simulink model "windEmulatorStep3"  (R2021a)
settings: Solver=ode4  StartTime=0.0  StopTime=inf  FixedStep=0.002  RelTol=1e-3
values from neighbouring files (symbols this model uses):
  ctrlModeSpeed = logical(false)    [initStep4.m]
  ctrlModeTorque = logical(true)    [initStep4.m]
  Dm_max = 40    [initStep4.m]
  EffMechMax = 0.93    [initStep4.m]
  EffMechMin = 0.79    [initStep4.m]
  FactorEff = psi2pa*cc2m3*(1/rev2rad)    (= 0.00109733470463)    [initStep4.m]
  genMaxTorque = 0.975*acs880RatedTorque    (= 78.48165)    [initStep4.m]
  Kdamping = -500    [OptimizationResultsLoad.m]
  Kpos = 0    [OptimizationResultsLoad.m]
  nPreDrop = 2900    [initStep4.m]
  nPreDropMin = 725    [initStep4.m]
  StatusWord = bitset(StatusWord,16)    [VFD_StatusWord.m]
  T = 4    [initStep4.m]
  wheelRadius = targetWaveBotVel/targetOmega    (= 0.00477464829276)    [initStep4.m]
undefined symbols (not defined in the file or in its folder): ACS880PILimLo, ACS880PILimUp, DiscIntNeverNeededParam, Gen_REF2_Max, Gen_SpeedScaling, minPressureRef, Motor_SpeedScaling, Motor_TorqueScaling, PressureControl, ratedTorque, rpm2rps, SpeedControl, speedScalingACS800, TorqueFieldbusScale, TorqueInputControl, TorqueRefMin
libraries: fl_lib x41, nesl_utility x24, slrealtimeethercatlib x21, sh_lib x16, cstblocks x4, simulink x3, pid_lib x3, sdl_lib x1, dspstat3 x1
(part 1 of 3)
settings Model: SimulationMode=external  Creator=SWEPT  LastModifiedBy=SWEPT
settings SolverCC: ConcurrentTasks=on  PositivePriorityOrder=on
settings OptimizationCC: BlockReduction=off  OptimizeBlockIOStorage=off
settings DebuggingCC: TasksWithSamePriorityMsg=none
settings HardwareCC: ProdBitPerLong=64  ProdLongLongMode=on  ProdHWDeviceType=Intel->x86-64 (Linux 64)
settings RTWCC: Description=Simulink Real-Time  SystemTargetFile=slrealtime.tlc  TemplateMakefile=slrealtime_default_tmf  RTWVerbose=off  Toolchain=Simulink Real-Time Toolchain  BuildConfiguration=Faster Runs  CodeExecutionProfiling=on  TargetLang=C++

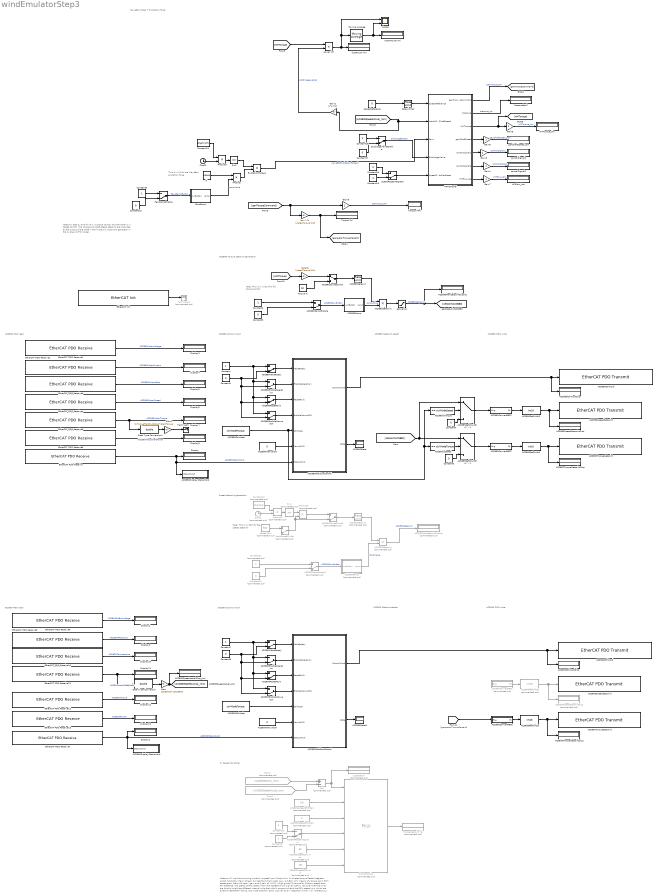
== system windEmulatorStep3 ==
  note: WaveBot Model + Excitation force
  note: PI Speed Controller
  note: Notes on PI:
      |
      | Input to summing junction is speed (rpm)
      | Output is in % of rated torque
      | Reset Integrator switch holds the I-Term at zero, but lets the P-Term pass.
      |
      | e.g., a P-Gain of 1 means 1% torque per 1 RPM speed error. Start with zero I gain and P gain of ~0.01, which gives 1% torque for 100rpm speed error.
      |
      | For reference, the speed control section from the ACS800 drive is given below. Not sure what the units are for this (might be different internal units than the % torque unit and the RPM speed unit, which are external (EtherCAT) facing. Also note that the I terms is given as an integration time in (s), whereas our integral term is a gain of the form Ki/s. The conversion should be: Ki = Kp/Ti. So to convert 2.5s with Kp = 10 gives Ki = 10/2.5 = 4.
      |
      | Jon undertook a re-tuning for the ACS880. This gave Kp = 5.84 and Ti = 0.33s. With this, Ki = 5.84/0.33 = 17.7.
      |
      | Start tuning Kp first, and then slowly bring Ki up to ~1-3 times Kp.
  note: Notes on Step 3:
      |
      | One drive is in torque control and the other is in speed control.
      |
      | The torque and shaft speed setpoint are produced as the output of the shaft in the hydraulic motor and generator in the hydraulic PTO model.
  note: ACS880 Torque setpoint generation
  note: ACS880 PDO write
  note: ASC880 Setpoint select
  note: Note: This is in units of % for torque control
  note: ACS880 Control Word
  note: ACS880 PDO read
  note: ACS800 PDO read
  note: ACS800 Control Word
  note: ASC800 Setpoint select
  note: ACS800 PDO write
  note: Speed setpoint generation
  note: Note: This is in RPM for the speed setpoint
  note: This is in (N) for the WaveBot excitation force
  ACS800ConvertREF1 : Subsystem  Commented=on  mask{EngineeringValue=Gen_SpeedScaling, FieldbusValue=20000}
      mask prompts: EngineeringValue "Engineering units nominal value:"; FieldbusValue "Fieldbus nominal value:"
  ACS800ConvertREF2 : Subsystem  mask{EngineeringValue=Gen_REF2_Max, FieldbusValue=10000}
      mask prompts: EngineeringValue "Engineering units nominal value:"; FieldbusValue "Fieldbus nominal value:"
  ACS800CtrlMode : Constant  Value=ctrlModeTorque  OutDataTypeStr=boolean
  ACS800CtrlWord : slrealtimeethercatlib/EtherCAT PDO Transmit  Priority=3  sig_name=Drive 2 (RECA-01 r2.07 and ACS800).RxPDO 1.ControlWord (Transparent)  sig_offset=384  sig_type=uint16  type_size=16  sig_dim=1  device_id=0  sample_time=0.002000
      settings: SourceProductBaseCode=XP
  ACS800CtrlWordDisp : Display
  ACS800DisplayStatusWord : Subsystem
  ACS800FieldbusControl : Subsystem
  ACS800ManualCW : Constant  Value=0  OutDataTypeStr=uint16
  ACS800Ramp : Stateflow chart  Commented=on  TreatAsAtomicUnit=on
  ACS800RampEnable : ManualSwitch  Commented=on  CurrentSetting=0
  ACS800RateLim : RateLimiter  Commented=on  RisingSlewLimit=10000  FallingSlewLimit=-10000  SampleTimeMode=inherited
  ACS800RawSetpointDisplay : Display  Commented=on
  ACS800Ref1Int16 : DataTypeConversion  Commented=on  OutDataTypeStr=int16
  ACS800Ref2Int16 : DataTypeConversion  OutDataTypeStr=int16
  ACS800ResetIntegrator : ManualSwitch  Commented=on  CurrentSetting=0
  ACS800Setpoint : Product  Commented=on
  ACS800SpeedCtrlIGain : Constant  Commented=on  Value=0
  ACS800SpeedCtrlLimLo : Constant  Commented=on  Value=-80
  ACS800SpeedCtrlLimUp : Constant  Commented=on  Value=80
  ACS800SpeedCtrlPGain : Constant  Commented=on  Value=0.6
  ACS800SpeedSetpoint : slrealtimeethercatlib/EtherCAT PDO Transmit  Priority=3  sig_name=Drive 2 (RECA-01 r2.07 and ACS800).RxPDO 1.REF1 (Speed)  sig_offset=400  sig_type=int16  type_size=16  sig_dim=1  device_id=0  sample_time=0.002000
      settings: SourceProductBaseCode=XP
  ACS800SpeedSetpointDisp : Display  Commented=on
  ACS800TorqueSetpoint : slrealtimeethercatlib/EtherCAT PDO Transmit  Priority=3  sig_name=Drive 2 (RECA-01 r2.07 and ACS800).RxPDO 1.REF2 (Torque)  sig_offset=416  sig_type=int16  type_size=16  sig_dim=1  device_id=0  sample_time=0.002000
      settings: SourceProductBaseCode=XP
  ACS800TorqueSetpointDisp : Display
  ACS880ConvertREF1 : Subsystem  mask{EngineeringValue=Motor_SpeedScaling, FieldbusValue=20000}
      mask prompts: EngineeringValue "Engineering units nominal value:"; FieldbusValue "Fieldbus nominal value:"
  ACS880ConvertREF2 : Subsystem  mask{EngineeringValue=Motor_TorqueScaling, FieldbusValue=10000}
      mask prompts: EngineeringValue "Engineering units nominal value:"; FieldbusValue "Fieldbus nominal value:"
  ACS880CtrlMode : Constant  Value=ctrlModeTorque  OutDataTypeStr=boolean
  ACS880CtrlWord : slrealtimeethercatlib/EtherCAT PDO Transmit  Priority=3  sig_name=Drive 1 (FECA-01 r1.31 and ACS880).RxPDO 1.ABB Drives Control Word  sig_offset=208  sig_type=uint16  type_size=16  sig_dim=1  device_id=0  sample_time=0.002000
      settings: SourceProductBaseCode=XP
  ACS880CtrlWordDisp : Display
  ACS880DisplayStatusWord : Subsystem
  ACS880FieldbusControl : Subsystem
  ACS880IsTorque : simulink/Logic and Bit Operations/Compare To Constant  relop===  const=ctrlModeSpeed  OutDataTypeStr=boolean
  ACS880ManualCW : Constant  Value=0  OutDataTypeStr=uint16
  ACS880Ramp : Stateflow chart  TreatAsAtomicUnit=on
  ACS880RampEnable : ManualSwitch  CurrentSetting=0
  ACS880RateLim : RateLimiter  RisingSlewLimit=10000  FallingSlewLimit=-10000  SampleTimeMode=inherited
  ACS880RawSetpointDisplay : Display
  ACS880Ref1Int16 : DataTypeConversion  OutDataTypeStr=int16
  ACS880Ref1Switch : Switch  Criteria=u2 > Threshold
  ACS880Ref2Int16 : DataTypeConversion  OutDataTypeStr=int16
  ACS880Ref2Switch : Switch  Criteria=u2 > Threshold
  ACS880Setpoint : Product
  ACS880SpeedActualDisp_rpm : Display
  ACS880SpeedSetpoint : slrealtimeethercatlib/EtherCAT PDO Transmit  Priority=3  sig_name=Drive 1 (FECA-01 r1.31 and ACS880).RxPDO 1.ABB Drives REF1  sig_offset=224  sig_type=int16  type_size=16  sig_dim=1  device_id=0  sample_time=0.002000
      settings: SourceProductBaseCode=XP
  ACS880SpeedSetpointDisp : Display
  ACS880TorqueSetpoint : slrealtimeethercatlib/EtherCAT PDO Transmit  Priority=3  sig_name=Drive 1 (FECA-01 r1.31 and ACS880).RxPDO 1.ABB Drives REF2  sig_offset=240  sig_type=int16  type_size=16  sig_dim=1  device_id=0  sample_time=0.002000
      settings: SourceProductBaseCode=XP
  ACS880TorqueSetpointDisp : Display
  ASC800EnableManualCW : ManualSwitch  CurrentSetting=0
  ASC800EnableOperation : ManualSwitch  CurrentSetting=0
  ASC800MakeReady : ManualSwitch  CurrentSetting=0
  ASC800ResetFault : ManualSwitch  CurrentSetting=0
  ASC800SourceSwitch : ManualSwitch  Commented=on  CurrentSetting=0
  ASC880EnableManualCW : ManualSwitch  CurrentSetting=0
  ASC880EnableOperation : ManualSwitch  CurrentSetting=0
  ASC880IsSpeed : simulink/Logic and Bit Operations/Compare To Constant  relop===  const=ctrlModeTorque  OutDataTypeStr=boolean
  ASC880MakeReady : ManualSwitch  CurrentSetting=0
  ASC880ResetFault : ManualSwitch  CurrentSetting=0
  ASC880SourceSwitch : ManualSwitch
  ASC880State : Display
  ASC880State1 : Display
  Add : Sum  Commented=on  Inputs=+-
  Clock1 : Clock  Commented=on
  Clock2 : Clock
  Constant{,2,5,7,16,19} (6 alike) : Constant
  Constant{1,3..4,6,8,15,17..18} (8 alike) : Constant  Value=0
  Constant10 : Constant  Commented=on  Value=0
  Constant11 : Constant  Commented=on
  Constant12 : Constant  Commented=on  Value=0
  Constant13 : Constant  Commented=on  Value=2*pi*0.2
  Constant14 : Constant  Value=2*pi*(1/T)
  Constant9 : Constant  Commented=on
  Data Type Conversion : DataTypeConversion  OutDataTypeStr=double
  Data Type Conversion1 : DataTypeConversion  OutDataTypeStr=double
  DischargeValveEnable : ManualSwitch  CurrentSetting=0
  Display{,1..13} (14 alike) : Display
  EtherCAT Init : slrealtimeethercatlib/EtherCAT Init  Priority=0  config_file=C:\Users\SWEPT\Desktop\Jorge\WIndTurbineEmulator\WindEmulatorFiles\ethercat\WindTurbineEmulator-03-24-2022.xml  device_id=0  pci_bus=0  pci_slot=0  pci_function=0  portnum=1  initstate=2  dctuning=0  enaDebug=0  enaDC=on  errLink=off  masterDbg=off  stateChgDbg=off  baseClock=off  masterCfg=off  logFile='c:\dbglog.txt'  sample_time=0.002000  DCMode=0
      settings: SourceProductBaseCode=XP
  EtherCAT PDO Receive : slrealtimeethercatlib/EtherCAT PDO Receive  Priority=2  sig_name=Drive 1 (FECA-01 r1.31 and ACS880).TxPDO 1.ABB Drives Status Word  sig_offset=208  sig_type=uint16  type_size=16  sig_dim=1  device_id=0  sample_time=0.002000
      settings: SourceProductBaseCode=XP
  EtherCAT PDO Receive1 : slrealtimeethercatlib/EtherCAT PDO Receive  Priority=2  sig_name=Drive 1 (FECA-01 r1.31 and ACS880).TxPDO 6.Calculated motor voltage  sig_offset=304  sig_type=int16  type_size=16  sig_dim=1  device_id=0  sample_time=0.002000
      settings: SourceProductBaseCode=XP
  EtherCAT PDO Receive10 : slrealtimeethercatlib/EtherCAT PDO Receive  Priority=2  sig_name=Drive 2 (RECA-01 r2.07 and ACS800).TxPDO 1.Converter Temperature  sig_offset=496  sig_type=int16  type_size=16  sig_dim=1  device_id=0  sample_time=0.002000
      settings: SourceProductBaseCode=XP
  EtherCAT PDO Receive11 : slrealtimeethercatlib/EtherCAT PDO Receive  Priority=2  sig_name=Drive 2 (RECA-01 r2.07 and ACS800).TxPDO 1.Actual Feedback (Transparent)  sig_offset=400  sig_type=int16  type_size=16  sig_dim=1  device_id=0  sample_time=0.002000
      settings: SourceProductBaseCode=XP
  EtherCAT PDO Receive12 : slrealtimeethercatlib/EtherCAT PDO Receive  Priority=2  sig_name=Drive 2 (RECA-01 r2.07 and ACS800).TxPDO 1.Torque  sig_offset=432  sig_type=int16  type_size=16  sig_dim=1  device_id=0  sample_time=0.002000
      settings: SourceProductBaseCode=XP
  EtherCAT PDO Receive13 : slrealtimeethercatlib/EtherCAT PDO Receive  Priority=2  sig_name=Drive 2 (RECA-01 r2.07 and ACS800).TxPDO 1.Power  sig_offset=448  sig_type=int16  type_size=16  sig_dim=1  device_id=0  sample_time=0.002000
      settings: SourceProductBaseCode=XP
  EtherCAT PDO Receive2 : slrealtimeethercatlib/EtherCAT PDO Receive  Priority=2  sig_name=Drive 1 (FECA-01 r1.31 and ACS880).TxPDO 6.Measured motor current  sig_offset=288  sig_type=int16  type_size=16  sig_dim=1  device_id=0  sample_time=0.002000
      settings: SourceProductBaseCode=XP
  EtherCAT PDO Receive3 : slrealtimeethercatlib/EtherCAT PDO Receive  Priority=2  sig_name=Drive 1 (FECA-01 r1.31 and ACS880).TxPDO 6.Estimated output frequency  sig_offset=272  sig_type=int16  type_size=16  sig_dim=1  device_id=0  sample_time=0.002000
      settings: SourceProductBaseCode=XP
  EtherCAT PDO Receive4 : slrealtimeethercatlib/EtherCAT PDO Receive  Priority=2  sig_name=Drive 1 (FECA-01 r1.31 and ACS880).TxPDO 6.Motor speed used  sig_offset=256  sig_type=int16  type_size=16  sig_dim=1  device_id=0  sample_time=0.002000
      settings: SourceProductBaseCode=XP
  EtherCAT PDO Receive5 : slrealtimeethercatlib/EtherCAT PDO Receive  Priority=2  sig_name=Drive 1 (FECA-01 r1.31 and ACS880).TxPDO 6.Motor torque  sig_offset=320  sig_type=int16  type_size=16  sig_dim=1  device_id=0  sample_time=0.002000
      settings: SourceProductBaseCode=XP
  EtherCAT PDO Receive6 : slrealtimeethercatlib/EtherCAT PDO Receive  Priority=2  sig_name=Drive 1 (FECA-01 r1.31 and ACS880).TxPDO 6.Estimated motor shaft power  sig_offset=336  sig_type=int16  type_size=16  sig_dim=1  device_id=0  sample_time=0.002000
      settings: SourceProductBaseCode=XP
  EtherCAT PDO Receive7 : slrealtimeethercatlib/EtherCAT PDO Receive  Priority=2  sig_name=Drive 2 (RECA-01 r2.07 and ACS800).TxPDO 1.Main StatusWord (Transparent)  sig_offset=384  sig_type=uint16  type_size=16  sig_dim=1  device_id=0  sample_time=0.002000
      settings: SourceProductBaseCode=XP
  EtherCAT PDO Receive8 : slrealtimeethercatlib/EtherCAT PDO Receive  Priority=2  sig_name=Drive 2 (RECA-01 r2.07 and ACS800).TxPDO 1.DC Bus Voltage  sig_offset=480  sig_type=int16  type_size=16  sig_dim=1  device_id=0  sample_time=0.002000
      settings: SourceProductBaseCode=XP
  EtherCAT PDO Receive9 : slrealtimeethercatlib/EtherCAT PDO Receive  Priority=2  sig_name=Drive 2 (RECA-01 r2.07 and ACS800).TxPDO 1.Frequency  sig_offset=464  sig_type=int16  type_size=16  sig_dim=1  device_id=0  sample_time=0.002000
      settings: SourceProductBaseCode=XP
  ExcitationForce_N : Product
  FexcRamp : Stateflow chart  TreatAsAtomicUnit=on
  FexcRampEnable : ManualSwitch  CurrentSetting=0
  From1 : From  Commented=on  GotoTag=ACS800SpeedActual_rpm
  From2 : From  Commented=on  GotoTag=speedSetpoint_rpm
  Gain : Gain  Gain=speedScalingACS800
  Gain1 : Gain  Gain=(1/TorqueFieldbusScale)*ratedTorque
  Gain2 : Gain  Gain=(2*pi)/60
  Gain{3..8} (6 alike) : Gain
  HMFlow_lpm : Display
  HMTorque_Nm : Display
  HPTOModel : Subsystem
  Moving Average : dspstat3/Moving Average  Method=Sliding window  ForgettingFactorPort=off  SpecifyWindowLength=on  WindowLength=20*500  ForgettingFactor=0.9  SimulateUsing=Code generation
  N : Constant  Value=15000
  "Nm -> %" : Gain  Gain=1/ratedTorque*100
  Nmto% : Gain  Gain=1/ratedTorque*100
  PID Controller : pid_lib/PID Controller  Commented=on  Controller=PI  Form=Parallel  TimeDomain=Discrete-time  UseExternalTs=off  SampleTime=-1  IntegratorMethod=Forward Euler  FilterMethod=Forward Euler  ControllerParametersSource=external  P=1  I=1  D=0  UseFilter=on  N=100  TunerSelectOption=Transfer Function Based (PID Tuner App)  InitialConditionSource=internal  InitialConditionForIntegrator=0  InitialConditionForFilter=0  DifferentiatorICPrevScaledInput=0  ExternalReset=level  TrackingMode=off  Kt=1  LimitOutput=on  SatLimitsSource=external  UpperSaturationLimit=inf  LowerSaturationLimit=-inf  LinearizeAsGain=on  AntiWindupMode=clamping  Kb=1  POutMin=[]  POutMax=[]  IOutMin=[]  IOutMax=[]  DOutMin=[]  DOutMax=[]  NOutMin=[]  NOutMax=[]  SumOutMin=[]  SumOutMax=[]  SaturationOutMin=[]  SaturationOutMax=[]  PParamMin=[]  PParamMax=[]  IParamMin=[]  IParamMax=[]  DParamMin=[]  DParamMax=[]  NParamMin=[]  NParamMax=[]  KbParamMin=[]  KbParamMax=[]  KtParamMin=[]  KtParamMax=[]  KbOutMin=[]  KbOutMax=[]  KtOutMin=[]  KtOutMax=[]  IntegratorOutMin=[]  IntegratorOutMax=[]  FilterOutMin=[]  FilterOutMax=[]  SumI1OutMin=[]  SumI1OutMax=[]  SumI2OutMin=[]  SumI2OutMax=[]  SumI3OutMin=[]  SumI3OutMax=[]  SumI4OutMin=[]  SumI4OutMax=[]  SumDOutMin=[]  SumDOutMax=[]  DifferentiatorOutMin=[]  DifferentiatorOutMax=[]  FilterDiffOutCoefMin=[]  FilterDiffOutCoefMax=[]  ReciprocalOutMin=[]  ReciprocalOutMax=[]  SumDenOutMin=[]  SumDenOutMax=[]  SumNumOutMin=[]  SumNumOutMax=[]  DivideOutMin=[]  DivideOutMax=[]  UdiffTsProdOutMin=[]  UdiffTsProdOutMax=[]  NTsProdOutMin=[]  NTsProdOutMax=[]  UintegralTsProdOutMin=[]  UintegralTsProdOutMax=[]  UngainTsProdOutMin=[]  UngainTsProdOutMax=[]  IntegratorContinuousStateAttributes=''  IntegratorStateMustResolveToSignalObject=off  IntegratorRTWStateStorageClass=Auto  FilterContinuousStateAttributes=''  FilterStateMustResolveToSignalObject=off  FilterRTWStateStorageClass=Auto  ParallelPVariant=ExternalParameters  IdealPVariant=Disabled  IVariant=ExternalParameters  DVariant=Disabled  IntegratorVariant=Discrete  SatVariant=External  AWVariant=DiscClampingParallel  PCopyVariant=Disabled  TRVariant=Disabled  FdbkBlocksVariant=Forward  IdealPFdbkVariant=Disabled  SatFdbkVariant=Disabled  DerivativeFilterVariant=Disabled  NVariant=Disabled  NCopyVariant=Disabled_SignalSpec  FilterICVariant=Disabled  IntegratorICVariant=InternalICs  ExternalResetVariant=ExternalReset  TRSumVariant=Passthrough  SumFdbkVariant=Disabled  SumVariant=Sum_PI  TsampFilterVariant=InternalTs  TsampNgainVariant=Passthrough  TsampIntegralVariant=Passthrough  ExternalSaturationOutDataTypeStr=Inherit: Same as second input
  Pressure[psi] : Display
  Product : Product
  Product2 : Product  Commented=on
  Product3 : Product  Commented=on
  Product4 : Product
  Rate Limiter : RateLimiter  RisingSlewLimit=50  FallingSlewLimit=-50  SampleTimeMode=inherited
  Saturation : Saturate  UpperLimit=ACS880PILimUp  LowerLimit=ACS880PILimLo
  Scope : Scope  NumInputPorts=2
  Sin1 : Trigonometry  Commented=on
  Sin2 : Trigonometry
  Speed RPM : Constant  Commented=on  Value=500
  SpeedError : Display  Commented=on
  SpeedReference : Constant  Value=0
  SpeedResetIntegrator : ManualSwitch  CurrentSetting=0
  Terminator : Terminator
  Terminator1 : Terminator  Commented=on
  Torque % : Constant  Value=10
  Torque (%) : Display
  Torque (Nm) : Display
  TorqueSetpoint (%) : Display  Commented=on
  controlSignal1 : Display
  controlSignal2 : Display
  dispPower (W) : Display
  genShaftSpeed_rpm : Display
  meanPower (W) : Display
  power (W) : Product
  shaftSpeedSwitch : ManualSwitch  Commented=on  CurrentSetting=0
  wires:
  EtherCAT Init/1 -> Terminator1/1
  ASC880EnableOperation/1 -> ACS880FieldbusControl/2(EnableOperation)
  ACS880ManualCW/1 -> ACS880FieldbusControl/6(ManualCW)
  ASC880ResetFault/1 -> ACS880FieldbusControl/3(ResetFault)
  ASC880MakeReady/1 -> ACS880FieldbusControl/1(MakeReady)
  ASC880EnableManualCW/1 -> ACS880FieldbusControl/4(EnableManualCW)
  Constant1/1 -> ASC880EnableManualCW/2, ASC880ResetFault/2, ASC880EnableOperation/2, ASC880MakeReady/2
  Constant/1 -> ASC880EnableManualCW/1, ASC880ResetFault/1, ASC880EnableOperation/1, ASC880MakeReady/1
  ACS880FieldbusControl/2(state) -> ASC880State/1
  EtherCAT PDO Receive1/1 -> Display3/1  "ACS880MotorVoltage"
  EtherCAT PDO Receive2/1 -> Display4/1  "ACS880MotorCurrent"
  EtherCAT PDO Receive3/1 -> Display5/1  "ACS880OutputFreq"
  EtherCAT PDO Receive4/1 -> Display6/1  "ACS880MotorSpeed"
  EtherCAT PDO Receive5/1 -> Display7/1, Data Type Conversion1/1  "ACS880MotorTorque"
  EtherCAT PDO Receive6/1 -> Display8/1  "ACS880MotorShaftPower"
  ACS880RampEnable/1 -> ACS880Ramp/1(runButton)  "ACS880RunButton"
  Constant3/1 -> ACS880RampEnable/2
  Constant2/1 -> ACS880RampEnable/1
  ACS880Ramp/1(ramp) -> ACS880Setpoint/2  "rampValue"
  ACS880Setpoint/1 -> Saturation/1
  ACS880RateLim/1 -> ACS880Setpoint/1
  ACS880ConvertREF1/1(Fb) -> ACS880Ref1Int16/1
  ACS880Ref1Int16/1 -> ACS880SpeedSetpointDisp/1, ACS880SpeedSetpoint/1
  ACS880Ref2Int16/1 -> ACS880TorqueSetpoint/1, ACS880TorqueSetpointDisp/1
  ACS880ConvertREF2/1(Fb) -> ACS880Ref2Int16/1
  ACS880CtrlMode/1 -> ACS880FieldbusControl/5(CtrlMode), ACS880IsTorque/1, ASC880IsSpeed/1
  EtherCAT PDO Receive/1 -> ACS880DisplayStatusWord/1(StatusWord), ACS880FieldbusControl/7(StatusWord), Display/1  "ACS880StatusWord"
  ACS880IsTorque/1 -> ACS880Ref1Switch/2
  [setpointACS880] -> ACS880Ref1Switch/1, ACS880Ref2Switch/1
  Constant4/1 -> ACS880Ref1Switch/3
  ASC880IsSpeed/1 -> ACS880Ref2Switch/2
  Constant6/1 -> ACS880Ref2Switch/3
  ACS880FieldbusControl/1(ControlWord) -> ACS880CtrlWordDisp/1, ACS880CtrlWord/1
  ACS880Ref1Switch/1 -> ACS880ConvertREF1/1(Eng)
  ACS880Ref2Switch/1 -> ACS880ConvertREF2/1(Eng)
  Torque %/1 -> ASC880SourceSwitch/2
  ASC880SourceSwitch/1 -> ACS880RateLim/1
  EtherCAT PDO Receive13/1 -> Display13/1  "ACS800Power"
  EtherCAT PDO Receive11/1 -> Data Type Conversion/1, Display11/1  "ACS800ActualFeedback"
  EtherCAT PDO Receive9/1 -> Display9/1  "ACS800Frequency"
  EtherCAT PDO Receive12/1 -> Display12/1  "ACS800Torque"
  EtherCAT PDO Receive10/1 -> Display10/1  "ACS800Temperature"
  EtherCAT PDO Receive8/1 -> Display2/1  "ACS800DcBusVoltage"
  ASC800EnableOperation/1 -> ACS800FieldbusControl/2(EnableOperation)
  ASC800ResetFault/1 -> ACS800FieldbusControl/3(ResetFault)
  ACS800ManualCW/1 -> ACS800FieldbusControl/6(ManualCW)
  EtherCAT PDO Receive7/1 -> ACS800DisplayStatusWord/1(StatusWord), ACS800FieldbusControl/7(StatusWord), Display1/1  "ACS800StatusWord"
  Constant7/1 -> ASC800EnableManualCW/1, ASC800ResetFault/1, ASC800EnableOperation/1, ASC800MakeReady/1
  ACS800FieldbusControl/2(state) -> ASC880State1/1
  Constant8/1 -> ASC800EnableManualCW/2, ASC800ResetFault/2, ASC800EnableOperation/2, ASC800MakeReady/2
  ASC800MakeReady/1 -> ACS800FieldbusControl/1(MakeReady)
  ASC800EnableManualCW/1 -> ACS800FieldbusControl/4(EnableManualCW)
  ACS800CtrlMode/1 -> ACS800FieldbusControl/5(CtrlMode)
  ACS800ConvertREF2/1(Fb) -> ACS800Ref2Int16/1
  ACS800Ref2Int16/1 -> ACS800TorqueSetpointDisp/1, ACS800TorqueSetpoint/1
  ACS800Ref1Int16/1 -> ACS800SpeedSetpoint/1, ACS800SpeedSetpointDisp/1
  ACS800ConvertREF1/1(Fb) -> ACS800Ref1Int16/1
  ACS800FieldbusControl/1(ControlWord) -> ACS800CtrlWordDisp/1, ACS800CtrlWord/1
  PID Controller/1 -> TorqueSetpoint (%)/1
  ASC800SourceSwitch/1 -> ACS800RateLim/1
  Product3/1 -> ASC800SourceSwitch/1
  Sin1/1 -> Product3/1
  ACS800RateLim/1 -> ACS800Setpoint/1
  ACS800Setpoint/1 -> ACS800RawSetpointDisplay/1  "ACS800Setpoint"
  Constant13/1 -> Product2/1
  Product2/1 -> Sin1/1
  Clock1/1 -> Product2/2
  ACS800Ramp/1(ramp) -> ACS800Setpoint/2  "rampValue"
  Constant11/1 -> ACS800RampEnable/1
  Constant12/1 -> ACS800RampEnable/2
  ACS800RampEnable/1 -> ACS800Ramp/1(runButton)  "ACS800RunButton"
  Gain/1 -> ACS880SpeedActualDisp_rpm/1, [ACS800SpeedActual_rpm]
  From2/1 -> Add/1
  From1/1 -> Add/2
  Add/1 -> SpeedError/1, PID Controller/1
  ACS800SpeedCtrlPGain/1 -> PID Controller/2
  ACS800SpeedCtrlIGain/1 -> PID Controller/3
  ACS800ResetIntegrator/1 -> PID Controller/4
  Constant9/1 -> ACS800ResetIntegrator/2
  Constant10/1 -> ACS800ResetIntegrator/1
  Data Type Conversion/1 -> Gain/1
  ACS800SpeedCtrlLimUp/1 -> PID Controller/5
  ACS800SpeedCtrlLimLo/1 -> PID Controller/6
  Product4/1 -> Sin2/1
  Clock2/1 -> Product4/2
  Constant14/1 -> Product4/1
  ExcitationForce_N/1 -> HPTOModel/3(Fexc)  "waveBotExcitationForce_N"
  [genTorqueCommand] -> Gain5/1, "Nm -> %"/1
  Sin2/1 -> ExcitationForce_N/1
  power (W)/1 -> Scope/1, Moving Average/1, dispPower (W)/1
  [ACS800SpeedActual_rpm] -> Gain2/1, HPTOModel/2(ActualGenShaftSpeed)
  Moving Average/1 -> Scope/2, meanPower (W)/1
  Saturation/1 -> [setpointACS880], ACS880RawSetpointDisplay/1  "ACS880Setpoint"
  Data Type Conversion1/1 -> Gain1/1
  HPTOModel/1(genTorqueCommand) -> [genTorqueCommand]  "genTorque_Nm"
  Constant5/1 -> FexcRampEnable/1
  Constant15/1 -> FexcRampEnable/2
  FexcRampEnable/1 -> FexcRamp/1(runButton)  "FexcRampButton"
  FexcRamp/1(ramp) -> Product/2  "rampValue"
  N/1 -> Product/1
  Product/1 -> ExcitationForce_N/2
  Speed RPM/1 -> shaftSpeedSwitch/1
  shaftSpeedSwitch/1 -> ASC800SourceSwitch/2, Product3/2
  HPTOModel/2(Pressure) -> Pressure[psi]/1  "pressure_psi"
  DischargeValveEnable/1 -> HPTOModel/4(DischargeValve)  "DischargeButton"
  Constant16/1 -> DischargeValveEnable/1
  Constant17/1 -> DischargeValveEnable/2
  Constant19/1 -> SpeedResetIntegrator/2
  Constant18/1 -> SpeedResetIntegrator/1
  SpeedResetIntegrator/1 -> HPTOModel/5(SpeedControllerReset)
  [generatorTorquePercent] -> ACS800ConvertREF2/1(Eng)
  "Nm -> %"/1 -> [generatorTorquePercent], Torque (%)/1
  SpeedReference/1 -> Rate Limiter/1
  HPTOModel/3(HMTorque) -> Gain6/1, [HMTorque]
  HPTOModel/4(genShaftSpeed) -> Gain8/1
  [HMTorque] -> Nmto%/1
  Nmto%/1 -> ASC880SourceSwitch/1
  Gain2/1 -> power (W)/2  "ptoOmega_radps"
  Gain1/1 -> Terminator/1
  HPTOModel/5(controlSignal1) -> Gain3/1
  HPTOModel/6(controlSignal2) -> Gain4/1
  HPTOModel/7(HMFlow_lps) -> Gain7/1
  Rate Limiter/1 -> HPTOModel/1(SpeedReference)
  Gain3/1 -> controlSignal1/1  "controlSignal1"
  Gain4/1 -> controlSignal2/1  "controlSignal2"
  Gain5/1 -> Torque (Nm)/1  "ptoTorque_Nm"
  Gain6/1 -> HMTorque_Nm/1  "HMTorque_Nm"
  [HMTorque] -> power (W)/1
  Gain7/1 -> HMFlow_lpm/1  "HMFlow_lpm"
  Gain8/1 -> genShaftSpeed_rpm/1  "genShaftSpeed_rpm"

== system windEmulatorStep3/ACS800ConvertREF1 ==
  Eng : Inport
  Constant EngineeringValue : Constant  Value=EngineeringValue
  Constant FieldbusValue : Constant  Value=FieldbusValue
  Product : Product  Inputs=**/
  Fb : Outport
  wires:
  Constant EngineeringValue/1 -> Product/3
  Constant FieldbusValue/1 -> Product/2
  Eng/1 -> Product/1
  Product/1 -> Fb/1

== system windEmulatorStep3/ACS800ConvertREF2 ==
  Eng : Inport
  Constant EngineeringValue : Constant  Value=EngineeringValue
  Constant FieldbusValue : Constant  Value=FieldbusValue
  Product : Product  Inputs=**/
  Fb : Outport
  wires:
  Constant EngineeringValue/1 -> Product/3
  Constant FieldbusValue/1 -> Product/2
  Eng/1 -> Product/1
  Product/1 -> Fb/1

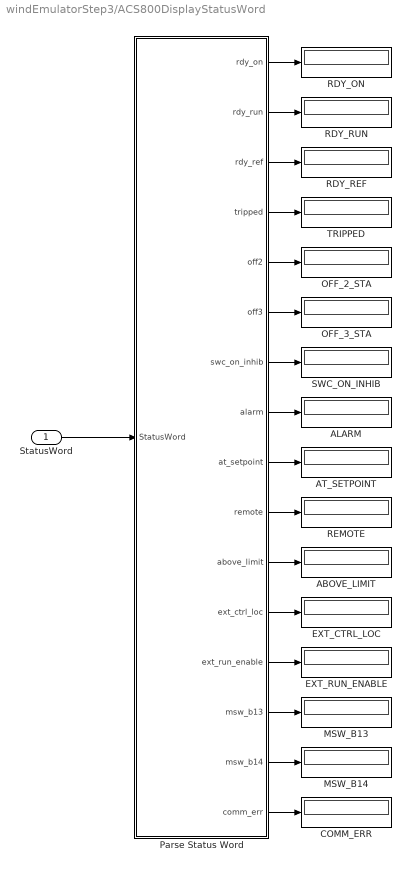
== system windEmulatorStep3/ACS800DisplayStatusWord ==
  StatusWord : Inport
  ABOVE_LIMIT : Display
  ALARM : Display
  AT_SETPOINT : Display
  COMM_ERR : Display
  EXT_CTRL_LOC : Display
  EXT_RUN_ENABLE : Display
  MSW_B13 : Display
  MSW_B14 : Display
  OFF_2_STA : Display
  OFF_3_STA : Display
  Parse Status Word : MATLAB Function  TreatAsAtomicUnit=on
  RDY_ON : Display
  RDY_REF : Display
  RDY_RUN : Display
  REMOTE : Display
  SWC_ON_INHIB : Display
  TRIPPED : Display
  wires:
  Parse Status Word/11(above_limit) -> ABOVE_LIMIT/1
  Parse Status Word/3(rdy_ref) -> RDY_REF/1
  Parse Status Word/16(comm_err) -> COMM_ERR/1
  Parse Status Word/15(msw_b14) -> MSW_B14/1
  Parse Status Word/14(msw_b13) -> MSW_B13/1
  Parse Status Word/8(alarm) -> ALARM/1
  Parse Status Word/2(rdy_run) -> RDY_RUN/1
  Parse Status Word/5(off2) -> OFF_2_STA/1
  Parse Status Word/12(ext_ctrl_loc) -> EXT_CTRL_LOC/1
  Parse Status Word/4(tripped) -> TRIPPED/1
  Parse Status Word/6(off3) -> OFF_3_STA/1
  Parse Status Word/1(rdy_on) -> RDY_ON/1
  Parse Status Word/9(at_setpoint) -> AT_SETPOINT/1
  Parse Status Word/7(swc_on_inhib) -> SWC_ON_INHIB/1
  Parse Status Word/13(ext_run_enable) -> EXT_RUN_ENABLE/1
  Parse Status Word/10(remote) -> REMOTE/1
  StatusWord/1 -> Parse Status Word/1(StatusWord)

== system windEmulatorStep3/ACS800FieldbusControl ==
  MakeReady : Inport
  EnableOperation : Inport  Port=2
  ResetFault : Inport  Port=3
  EnableManualCW : Inport  Port=4
  CtrlMode : Inport  Port=5
  ManualCW : Inport  Port=6  OutDataTypeStr=uint16
  StatusWord : Inport  Port=7
  ABB Fieldbus Control : Stateflow chart  TreatAsAtomicUnit=on
  Switch1 : Switch  Criteria=u2 ~= 0
  ControlWord : Outport
  state : Outport  Port=2
  wires:
  EnableOperation/1 -> ABB Fieldbus Control/1(EnableOperation)
  ManualCW/1 -> Switch1/1
  MakeReady/1 -> ABB Fieldbus Control/2(MakeReady)
  ABB Fieldbus Control/1(ControlWord) -> Switch1/3
  ResetFault/1 -> ABB Fieldbus Control/3(ResetFault)
  Switch1/1 -> ControlWord/1
  EnableManualCW/1 -> Switch1/2
  StatusWord/1 -> ABB Fieldbus Control/4(StatusWord)
  ABB Fieldbus Control/2(state) -> state/1
  CtrlMode/1 -> ABB Fieldbus Control/5(cwEXT_CTRL_LOC)

== system windEmulatorStep3/ACS880ConvertREF1 ==
  Eng : Inport
  Constant EngineeringValue : Constant  Value=EngineeringValue
  Constant FieldbusValue : Constant  Value=FieldbusValue
  Product : Product  Inputs=**/
  Fb : Outport
  wires:
  Product/1 -> Fb/1
  Eng/1 -> Product/1
  Constant FieldbusValue/1 -> Product/2
  Constant EngineeringValue/1 -> Product/3

== system windEmulatorStep3/ACS880ConvertREF2 ==
  Eng : Inport
  Constant EngineeringValue : Constant  Value=EngineeringValue
  Constant FieldbusValue : Constant  Value=FieldbusValue
  Product : Product  Inputs=**/
  Fb : Outport
  wires:
  Product/1 -> Fb/1
  Eng/1 -> Product/1
  Constant FieldbusValue/1 -> Product/2
  Constant EngineeringValue/1 -> Product/3

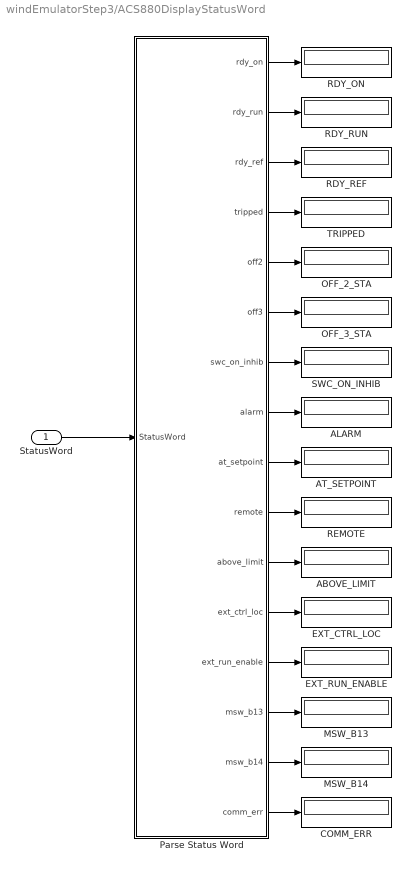
== system windEmulatorStep3/ACS880DisplayStatusWord ==
  StatusWord : Inport
  ABOVE_LIMIT : Display
  ALARM : Display
  AT_SETPOINT : Display
  COMM_ERR : Display
  EXT_CTRL_LOC : Display
  EXT_RUN_ENABLE : Display
  MSW_B13 : Display
  MSW_B14 : Display
  OFF_2_STA : Display
  OFF_3_STA : Display
  Parse Status Word : MATLAB Function  TreatAsAtomicUnit=on
  RDY_ON : Display
  RDY_REF : Display
  RDY_RUN : Display
  REMOTE : Display
  SWC_ON_INHIB : Display
  TRIPPED : Display
  wires:
  Parse Status Word/11(above_limit) -> ABOVE_LIMIT/1
  Parse Status Word/3(rdy_ref) -> RDY_REF/1
  Parse Status Word/16(comm_err) -> COMM_ERR/1
  Parse Status Word/15(msw_b14) -> MSW_B14/1
  Parse Status Word/14(msw_b13) -> MSW_B13/1
  Parse Status Word/8(alarm) -> ALARM/1
  Parse Status Word/2(rdy_run) -> RDY_RUN/1
  Parse Status Word/5(off2) -> OFF_2_STA/1
  Parse Status Word/12(ext_ctrl_loc) -> EXT_CTRL_LOC/1
  Parse Status Word/4(tripped) -> TRIPPED/1
  Parse Status Word/6(off3) -> OFF_3_STA/1
  Parse Status Word/1(rdy_on) -> RDY_ON/1
  Parse Status Word/9(at_setpoint) -> AT_SETPOINT/1
  Parse Status Word/7(swc_on_inhib) -> SWC_ON_INHIB/1
  Parse Status Word/13(ext_run_enable) -> EXT_RUN_ENABLE/1
  Parse Status Word/10(remote) -> REMOTE/1
  StatusWord/1 -> Parse Status Word/1(StatusWord)

== system windEmulatorStep3/ACS880FieldbusControl ==
  MakeReady : Inport
  EnableOperation : Inport  Port=2
  ResetFault : Inport  Port=3
  EnableManualCW : Inport  Port=4
  CtrlMode : Inport  Port=5
  ManualCW : Inport  Port=6  OutDataTypeStr=uint16
  StatusWord : Inport  Port=7
  ABB Fieldbus Control : Stateflow chart  TreatAsAtomicUnit=on
  Switch1 : Switch  Criteria=u2 ~= 0
  ControlWord : Outport
  state : Outport  Port=2
  wires:
  EnableOperation/1 -> ABB Fieldbus Control/1(EnableOperation)
  ManualCW/1 -> Switch1/1
  MakeReady/1 -> ABB Fieldbus Control/2(MakeReady)
  ABB Fieldbus Control/1(ControlWord) -> Switch1/3
  ResetFault/1 -> ABB Fieldbus Control/3(ResetFault)
  Switch1/1 -> ControlWord/1
  EnableManualCW/1 -> Switch1/2
  StatusWord/1 -> ABB Fieldbus Control/4(StatusWord)
  ABB Fieldbus Control/2(state) -> state/1
  CtrlMode/1 -> ABB Fieldbus Control/5(cwEXT_CTRL_LOC)

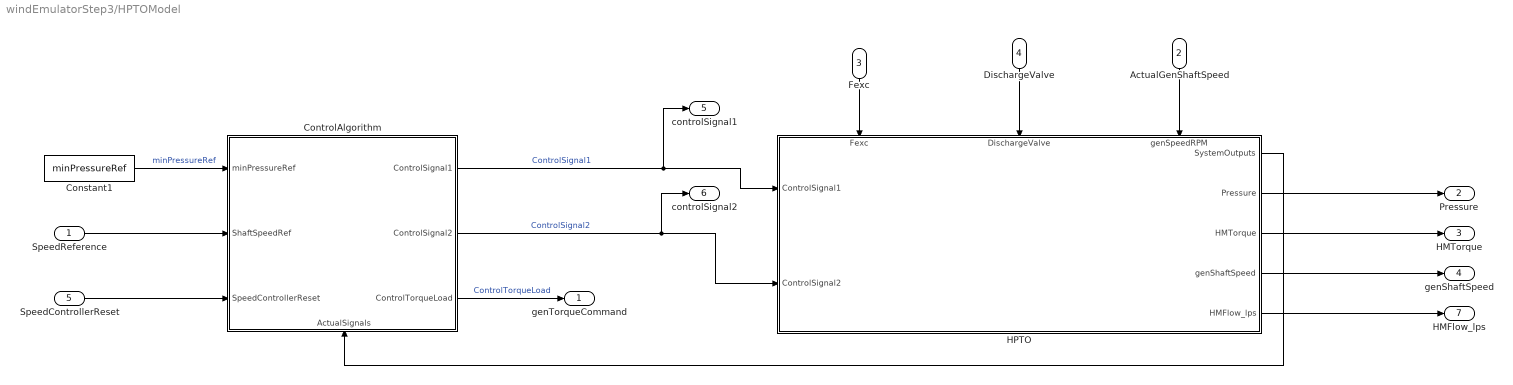
== system windEmulatorStep3/HPTOModel ==
  SpeedReference : Inport
  ActualGenShaftSpeed : Inport  Port=2
  Fexc : Inport  Port=3
  DischargeValve : Inport  Port=4
  SpeedControllerReset : Inport  Port=5
  Constant1 : Constant  Value=minPressureRef
  ControlAlgorithm : Subsystem
      settings: PortSchema="{\"entries\":[{\"content\":{\"sides\":[{\"content\":{\"connectorIds\":[\"In1\",\"In2\",\"In3\"]},\"type\":\"ConnectorPlacement.EquallySpacedRectSide\",\"uuid\":\"67adeffe-a398-49a8-b4a5-c43e48a316d9\"},{\"content\":{\"connectorIds\":[\"Out1\",\"Out2\",\"Out3\"],\"side\":\"RIGHT\"},\"type\":\"ConnectorPlacement.EquallySpacedRectSide\",\"uuid\":\"a2794d83-d293-4f11-b47e-435bf1d282f7\"},{\"content\":{\"connectorIds\":[],\"side\":\"TOP\"},\"type\":\"ConnectorPlacement.EquallySpacedRectSide\",\"uuid\":\"bb9f1178-f133-4eb3-bddb-bcb3a714b020\"},{\"content\":{\"connectorIds\":[\"In4\"],\"side\":\"BOTTOM\"},\"type\":\"ConnectorPlacement.EquallySpacedRectSide\",\"uuid\":\"388d2827-2454-4d01-b75f-f317c9ccd7ab\"}]},\"type\":\"ConnectorPlacement.EquallySpacedConnector\",\"uuid\":\"ef44af23-246a-43fe-a184-a2d38abebfbf\"}],\"packageUris\":[\"http://schema.mathworks.com/mf0/Connector/R2020b\"],\"version\":\"1.0\"}"
  HPTO : Subsystem
      settings: PortSchema="{\"entries\":[{\"content\":{\"sides\":[{\"content\":{\"connectorIds\":[\"In1\",\"In2\"]},\"type\":\"ConnectorPlacement.EquallySpacedRectSide\",\"uuid\":\"8fa4c7ba-45c7-41ba-9bcd-58cbee0318ba\"},{\"content\":{\"connectorIds\":[\"Out1\",\"Out2\",\"Out3\",\"Out4\",\"Out5\"],\"side\":\"RIGHT\"},\"type\":\"ConnectorPlacement.EquallySpacedRectSide\",\"uuid\":\"a23e9dd6-a871-47ae-a82a-10ea55782587\"},{\"content\":{\"connectorIds\":[\"In3\",\"In4\",\"In5\"],\"side\":\"TOP\"},\"type\":\"ConnectorPlacement.EquallySpacedRectSide\",\"uuid\":\"238aec0c-a47f-4ecc-bf69-7ee7f3fea80c\"}]},\"type\":\"ConnectorPlacement.EquallySpacedConnector\",\"uuid\":\"c89831dd-0ad8-4547-8547-63f84e5efa4b\"}],\"packageUris\":[\"http://schema.mathworks.com/mf0/Connector/R2020b\"],\"version\":\"1.0\"}"
  genTorqueCommand : Outport
  Pressure : Outport  Port=2
  HMTorque : Outport  Port=3
  genShaftSpeed : Outport  Port=4
  controlSignal1 : Outport  Port=5
  controlSignal2 : Outport  Port=6
  HMFlow_lps : Outport  Port=7
  wires:
  HPTO/1(SystemOutputs) -> ControlAlgorithm/4(ActualSignals)
  ControlAlgorithm/1(ControlSignal1) -> controlSignal1/1, HPTO/1(ControlSignal1)  "ControlSignal1"
  Constant1/1 -> ControlAlgorithm/1(minPressureRef)  "minPressureRef"
  ControlAlgorithm/2(ControlSignal2) -> controlSignal2/1, HPTO/2(ControlSignal2)  "ControlSignal2"
  Fexc/1 -> HPTO/3(Fexc)
  ActualGenShaftSpeed/1 -> HPTO/5(genSpeedRPM)
  HPTO/2(Pressure) -> Pressure/1
  ControlAlgorithm/3(ControlTorqueLoad) -> genTorqueCommand/1  "ControlTorqueLoad"
  DischargeValve/1 -> HPTO/4(DischargeValve)
  SpeedControllerReset/1 -> ControlAlgorithm/3(SpeedControllerReset)
  SpeedReference/1 -> ControlAlgorithm/2(ShaftSpeedRef)
  HPTO/3(HMTorque) -> HMTorque/1
  HPTO/4(genShaftSpeed) -> genShaftSpeed/1
  HPTO/5(HMFlow_lps) -> HMFlow_lps/1

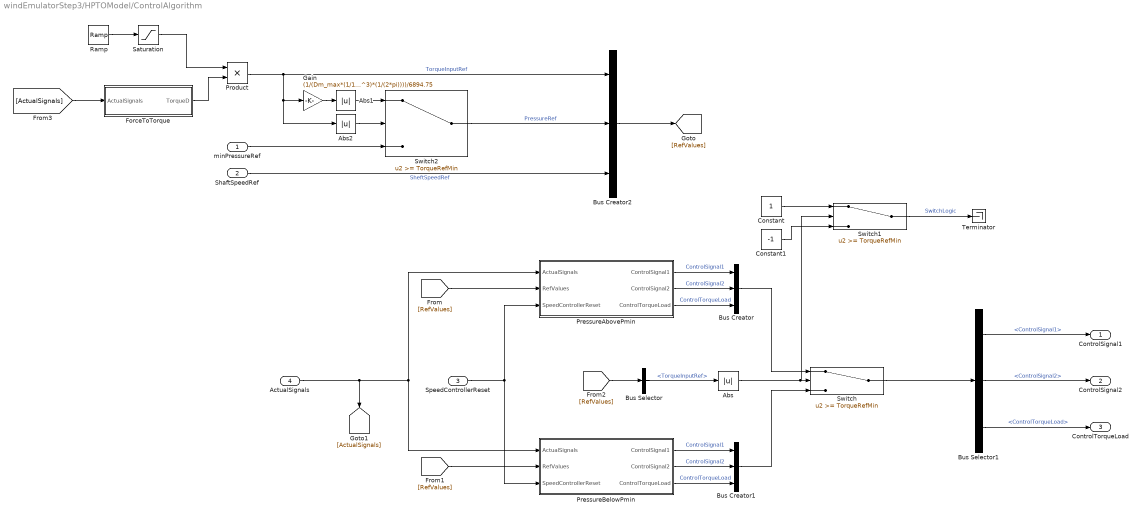
== system windEmulatorStep3/HPTOModel/ControlAlgorithm ==
  minPressureRef : Inport
  ShaftSpeedRef : Inport  Port=2
  SpeedControllerReset : Inport  Port=3
  ActualSignals : Inport  Port=4
  Abs : Abs
  Abs1 : Abs
  Abs2 : Abs
  Bus Creator : BusCreator  Inputs=3
  Bus Creator1 : BusCreator  Inputs=3
  Bus Creator2 : BusCreator  Inputs=3
  Bus Selector : BusSelector  OutputSignals=TorqueInputRef
  Bus Selector1 : BusSelector  OutputSignals=ControlSignal1,ControlSignal2,ControlTorqueLoad
  Constant : Constant
  Constant1 : Constant  Value=-1
  ForceToTorque : Subsystem
  Gain : Gain  Gain=(1/(Dm_max*(1/100^3)*(1/(2*pi))))/6894.75
  PressureAbovePmin : Subsystem
  PressureBelowPmin : Subsystem
  Product : Product
  Ramp : simulink/Sources/Ramp  slope=1/10  start=10  InitialOutput=0
  Saturation : Saturate  UpperLimit=1  LowerLimit=0
  Switch : Switch  Threshold=TorqueRefMin
  Switch1 : Switch  Threshold=TorqueRefMin
  Switch2 : Switch  Threshold=TorqueRefMin
  Terminator : Terminator
  ControlSignal1 : Outport
  ControlSignal2 : Outport  Port=2
  ControlTorqueLoad : Outport  Port=3
  wires:
  ActualSignals/1 -> [ActualSignals], PressureAbovePmin/1(ActualSignals), PressureBelowPmin/1(ActualSignals)
  PressureAbovePmin/1(ControlSignal1) -> Bus Creator/1  "ControlSignal1"
  PressureAbovePmin/2(ControlSignal2) -> Bus Creator/2  "ControlSignal2"
  PressureAbovePmin/3(ControlTorqueLoad) -> Bus Creator/3  "ControlTorqueLoad"
  Bus Creator/1 -> Switch/1
  PressureBelowPmin/1(ControlSignal1) -> Bus Creator1/1  "ControlSignal1"
  PressureBelowPmin/2(ControlSignal2) -> Bus Creator1/2  "ControlSignal2"
  PressureBelowPmin/3(ControlTorqueLoad) -> Bus Creator1/3  "ControlTorqueLoad"
  Bus Creator1/1 -> Switch/3
  Bus Selector1/1 -> ControlSignal1/1  "<ControlSignal1>"
  Bus Selector1/2 -> ControlSignal2/1  "<ControlSignal2>"
  Bus Selector1/3 -> ControlTorqueLoad/1  "<ControlTorqueLoad>"
  Product/1 -> Bus Creator2/1, Abs2/1, Gain/1  "TorqueInputRef"
  ShaftSpeedRef/1 -> Bus Creator2/3  "SheftSpeedRef"
  Bus Creator2/1 -> [RefValues]
  [RefValues] -> PressureAbovePmin/2(RefValues)
  [RefValues] -> PressureBelowPmin/2(RefValues)
  [RefValues] -> Bus Selector/1
  Bus Selector/1 -> Abs/1  "<TorqueInputRef>"
  Abs/1 -> Switch1/2, Switch/2
  Constant/1 -> Switch1/1
  Constant1/1 -> Switch1/3
  Switch1/1 -> Terminator/1  "SwitchLogic"
  Gain/1 -> Abs1/1
  Abs1/1 -> Switch2/1
  minPressureRef/1 -> Switch2/3
  Abs2/1 -> Switch2/2
  Switch2/1 -> Bus Creator2/2  "PressureRef"
  Saturation/1 -> Product/1
  Ramp/1 -> Saturation/1
  [ActualSignals] -> ForceToTorque/1(ActualSignals)
  ForceToTorque/1(TorqueD) -> Product/2
  Switch/1 -> Bus Selector1/1
  SpeedControllerReset/1 -> PressureAbovePmin/3(SpeedControllerReset), PressureBelowPmin/3(SpeedControllerReset)
